simulink model "jpp_dc_motor_regen_example2"  (R2016a)
settings: Solver=VariableStepAuto  StartTime=0.0  StopTime=tmax  FixedStep=.00001  RelTol=1e-3
values from neighbouring files (symbols this model uses):
  A = [ -R/L, -Kb/L ... (first row only)    [dc_motor_params_for_simulink.m]
  B = [1/L ... (first row only)    [dc_motor_params_for_simulink.m]
  C = eye(2)    [dc_motor_params_for_simulink.m]
  D = zeros(2,1)    [dc_motor_params_for_simulink.m]
  thresOff = .95*iss1    [dc_motor_params_for_simulink.m]
  thresOn = 0    [dc_motor_params_for_simulink.m]
  wss = xss(2)    [dc_motor_params_for_simulink.m]
settings Model: Creator=justin  LastModifiedBy=justin

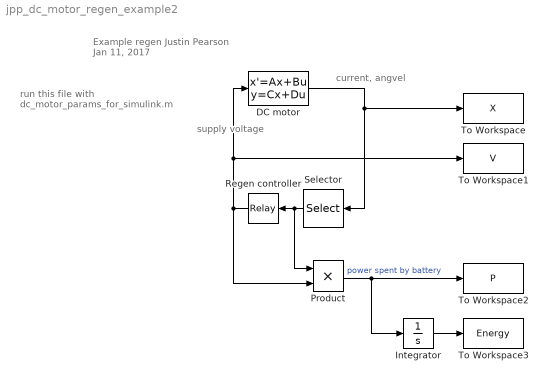
== system jpp_dc_motor_regen_example2 ==
  note: supply
      | voltage
  note: current, angvel
  note: run this file with
      | dc_motor_params_for_simulink.m
  note: Example regen
      | Justin Pearson
      | Jan 11, 2017
  DC motor : StateSpace  A=A  B=B  C=C  D=D  X0=[0;wss]
  Integrator : Integrator
  Product : Product
  Regen controller : Relay  OnSwitchValue=thresOn  OffSwitchValue=thresOff  OnOutputValue=voltOn  OffOutputValue=voltOff
  Selector : Selector  InputPortWidth=2  IndexOptions=Index vector (dialog)  Indices=[1]  OutputSizes=1
  To Workspace : ToWorkspace  VariableName=X  SaveFormat=Timeseries  SampleTime=-1
  To Workspace1 : ToWorkspace  VariableName=V  SaveFormat=Timeseries  SampleTime=-1
  To Workspace2 : ToWorkspace  VariableName=P  SaveFormat=Timeseries  SampleTime=-1
  To Workspace3 : ToWorkspace  VariableName=Energy  SaveFormat=Timeseries  SampleTime=-1
  wires:
  DC motor/1 -> Selector/1, To Workspace/1
  Regen controller/1 -> Product/2, DC motor/1, To Workspace1/1
  Selector/1 -> Product/1, Regen controller/1
  Product/1 -> Integrator/1, To Workspace2/1  "power spent by battery"
  Integrator/1 -> To Workspace3/1
